simulink model "vaja_04"  (R2020a)
settings: Solver=VariableStepAuto  StartTime=0.0  StopTime=1  RelTol=1e-3
settings Model: Creator=selmac  LastModifiedBy=selmac

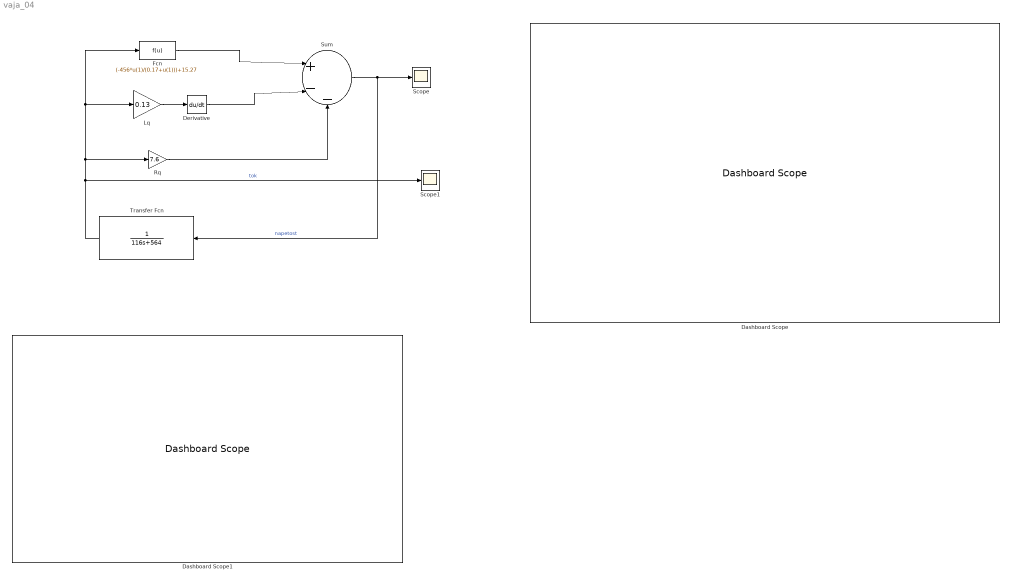
== system vaja_04 ==
  Dashboard Scope : DashboardScope  Ymin=0  Ymax=400
  Dashboard Scope1 : DashboardScope  Ymin=0  Ymax=0.8
  Derivative : Derivative
  Fcn : Fcn  Expr=(-456*u(1)/(0.17+u(1)))+15.27
  Lq : Gain  Gain=0.13
  Rq : Gain  Gain=7.6
  Scope : Scope
  Scope1 : Scope
  Sum : Sum  Inputs=|+--
  Transfer Fcn : TransferFcn  Denominator=[116 564]
  wires:
  Fcn/1 -> Sum/1
  Lq/1 -> Derivative/1
  Derivative/1 -> Sum/2
  Rq/1 -> Sum/3
  Sum/1 -> Transfer Fcn/1, Scope/1  "napetost"
  Transfer Fcn/1 -> Scope1/1, Rq/1, Lq/1, Fcn/1  "tok"
